simulink model "PannelTest"  (R2022b)
settings: Solver=FixedStepAuto  StartTime=0.0  StopTime=102  FixedStep=0.001  RelTol=1e-3
model workspace (MAT data in the model file):
  Manual_Auto = Simulink.Parameter
  Manual_Auto.Value = 0
  Manual_Auto.DataType = 'auto'
  Manual_Auto.Complexity = 'real'
  Manual_Auto.Dimensions = [1 1]
  Pattern = Simulink.Parameter
  Pattern.Value = 0
  Pattern.DataType = 'auto'
  Pattern.Complexity = 'real'
  Pattern.Dimensions = [1 1]
  Pause_Start = Simulink.Parameter
  Pause_Start.Value = 0
  Pause_Start.DataType = 'auto'
  Pause_Start.Complexity = 'real'
  Pause_Start.Dimensions = [1 1]
  Stop = Simulink.Parameter
  Stop.Value = 0
  Stop.DataType = 'auto'
  Stop.Complexity = 'real'
  Stop.Dimensions = [1 1]
  Unlock_Lock = Simulink.Parameter
  Unlock_Lock.Value = 0
  Unlock_Lock.DataType = 'auto'
  Unlock_Lock.Complexity = 'real'
  Unlock_Lock.Dimensions = [1 1]
undefined symbols (not defined in the file or in its folder): DiscIntNeverNeededParam
(part 1 of 3)
settings Model: Creator=My-Dell-PC  LastModifiedBy=My-Dell-PC

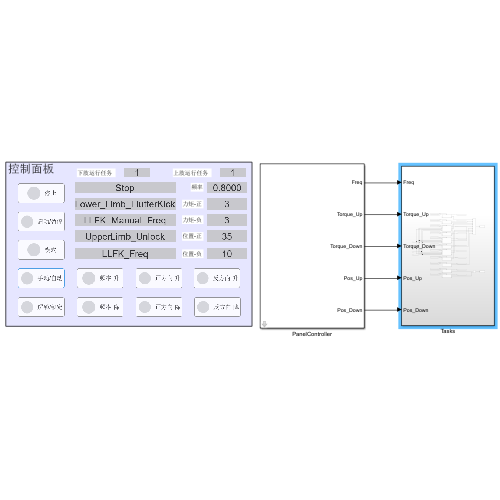
[thumbnail: Simulink's stored preview of the top-level diagram]
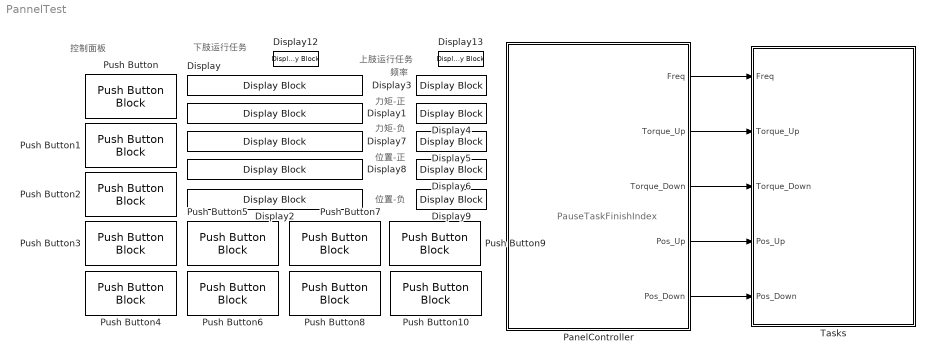
== system PannelTest ==
  note: PauseTaskFinishIndex
  note: 频率
  note: 控制面板
  note: 力矩-正
  note: 力矩-负
  note: 位置-正
  note: 位置-负
  note: 下肢运行任务
  note: 上肢运行任务
  Display{,1..9,12..13} (12 alike) : DisplayBlock  LabelPosition=Hide  Transparency=1
  PanelController : Subsystem  mask{LLFK_Freq_init=0.8, LLB_Freq_init=0.8, LLW_Freq_init=0.8, LLFK_Torque_Up_init=3, LLB_Torque_Up_init=3, LLW_Torque_Up_init=3, LLFK_Torque_Down_init=3, LLB_Torque_Down_init=3, LLW_Torque_Down_init=4.920, LLFK_Pos_Up_init=35, LLB_Pos_Up_init=35, LLW_Pos_Up_init=35, LLFK_Pos_Down_init=10, LLB_Pos_Down_init=10, LLW_Pos_Down_init=10}
      mask prompts: LLFK_Freq_init "LLFK_Freq_init (Hz)"; LLB_Freq_init "LLB_Freq_init (Hz)"; LLW_Freq_init "LLW_Freq_init (Hz)"; LLFK_Torque_Up_init "LLFK_Torque_Up_init (A)"; LLB_Torque_Up_init "LLB_Torque_Up_init (A)"; LLW_Torque_Up_init "LLW_Torque_Up_init (A)"; LLFK_Torque_Down_init "LLFK_Torque_Down_init (A)"; LLB_Torque_Down_init "LLB_Torque_Down_init (A)"; LLW_Torque_Down_init "LLW_Torque_Down_init (A)"; LLFK_Pos_Up_init "LLFK_Pos_Up_init (Degree)"; LLB_Pos_Up_init "LLB_Pos_Up_init (Degree)"; LLW_Pos_Up_init "LLW_Pos_Up_init (Degree)"; LLFK_Pos_Down_init "LLFK_Pos_Down_init (Degree)"; LLB_Pos_Down_init "LLB_Pos_Down_init (Degree)"; LLW_Pos_Down_init "LLW_Pos_Down_init (Degree)"
      mask DialogControl ParameterGroupVar Prompt: Freq_Init
      mask DialogControl Container3 Prompt: Torque_Up_Init
      mask DialogControl Container4 Prompt: Torque_Down_Init
      mask DialogControl Container5 Prompt: Pos_Up_init (Degree)
      mask DialogControl Container6 Prompt: Pos_Down_init (Degree)
  Push Button : PushButtonBlock  ButtonText=停止  Icon=Circle  IconColor=On  OffValue=0.000000
  Push Button1 : PushButtonBlock  ButtonText=启动/暂停  Icon=Circle  IconColor=On  OffValue=0.000000
  Push Button10 : PushButtonBlock  ButtonText=反方向-降  Icon=Circle  IconColor=On  OffValue=0.000000
  Push Button2 : PushButtonBlock  ButtonText=模式  Icon=Circle  IconColor=On  OffValue=0.000000
  Push Button3 : PushButtonBlock  ButtonText=手动/自动  Icon=Circle  IconColor=On  OffValue=0.000000
  Push Button4 : PushButtonBlock  ButtonText=解锁/锁定  Icon=Circle  IconColor=On  OffValue=0.000000
  Push Button5 : PushButtonBlock  ButtonText=频率-升  Icon=Circle  IconColor=On  OffValue=0.000000
  Push Button6 : PushButtonBlock  ButtonText=频率-降  Icon=Circle  IconColor=On  OffValue=0.000000
  Push Button7 : PushButtonBlock  ButtonText=正方向-升  Icon=Circle  IconColor=On  OffValue=0.000000
  Push Button8 : PushButtonBlock  ButtonText=正方向-降  Icon=Circle  IconColor=On  OffValue=0.000000
  Push Button9 : PushButtonBlock  ButtonText=反方向-升  Icon=Circle  IconColor=On  OffValue=0.000000
  Tasks : Subsystem
  wires:
  PanelController/1(Freq) -> Tasks/1(Freq)
  PanelController/2(Torque_Up) -> Tasks/2(Torque_Up)
  PanelController/3(Torque_Down) -> Tasks/3(Torque_Down)
  PanelController/4(Pos_Up) -> Tasks/4(Pos_Up)
  PanelController/5(Pos_Down) -> Tasks/5(Pos_Down)

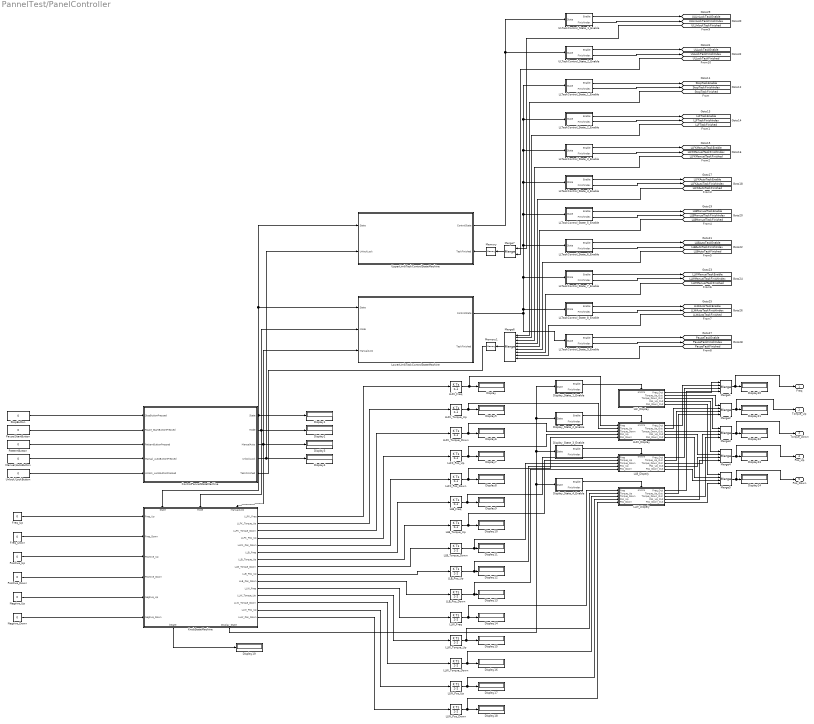
== system PannelTest/PanelController ==
  ControlPannelStateMachine : Stateflow chart  TreatAsAtomicUnit=on
      settings: PortSchema="{\"entries\":[{\"content\":{\"sides\":[{\"content\":{\"connectorIds\":[\"In2\",\"In3\",\"In4\",\"In5\",\"In6\"]},\"type\":\"ConnectorPlacement.EquallySpacedRectSide\",\"uuid\":\"eab411cf-4b6a-48c6-b596-b66f8c420e7c\"},{\"content\":{\"connectorIds\":[\"Out1\",\"Out2\",\"Out3\",\"Out4\",\"In1\"],\"side\":\"RIGHT\"},\"type\":\"ConnectorPlacement.EquallySpacedRectSide\",\"uuid\":\"e0e09f46-7c1c-4140-8220-034119073277\"},{\"content\":{\"connectorIds\":[],\"side\":\"TOP\"},\"type\":\"ConnectorPlacement.EquallySpacedRectSide\",\"uuid\":\"ed6bf201-0ea3-4e7c-82a9-322f02ea728a\"}]},\"type\":\"ConnectorPlacement.EquallySpacedConnector\",\"uuid\":\"aa71b69e-402d-40b0-a3fd-c9400a9adadc\"}],\"packageUris\":[\"http://schema.mathworks.com/mf0/Connector/R2020b\"],\"version\":\"1.0\"}"
  Display{,1..24} (25 alike) : Display
  Display_State_1_Enable : Subsystem  mask{TaskIndex=1}
  Display_State_2_Enable : Subsystem  mask{TaskIndex=2}
  Display_State_3_Enable : Subsystem  mask{TaskIndex=3}
  Display_State_4_Enable : Subsystem  mask{TaskIndex=4}
  Freq_Down : Constant  Value=0
  Freq_Up : Constant  Value=0
  KnobStateMachine : Stateflow chart  TreatAsAtomicUnit=on
      settings: PortSchema="{\"entries\":[{\"content\":{\"sides\":[{\"content\":{\"connectorIds\":[\"In1\",\"In2\",\"In3\",\"In4\",\"In5\",\"In6\"]},\"type\":\"ConnectorPlacement.EquallySpacedRectSide\",\"uuid\":\"78a56fe3-ceb0-42ee-90bc-aa39a12c9afb\"},{\"content\":{\"connectorIds\":[\"Out5\",\"Out3\",\"Out4\",\"Out6\",\"Out7\",\"Out8\",\"Out9\",\"Out10\",\"Out11\",\"Out12\",\"Out13\",\"Out14\",\"Out15\",\"Out16\",\"Out17\"],\"side\":\"RIGHT\"},\"type\":\"ConnectorPlacement.EquallySpacedRectSide\",\"uuid\":\"7553af84-a921-4f96-ace4-e42d4d568d32\"},{\"content\":{\"connectorIds\":[\"In7\",\"In8\",\"In9\"],\"side\":\"TOP\"},\"type\":\"ConnectorPlacement.EquallySpacedRectSide\",\"uuid\":\"299fd0e5-cc5b-4534-8b50-a134eaae2b47\"},{\"content\":{\"connectorIds\":[\"Out1\",\"Out2\"],\"side\":\"BOTTOM\"},\"type\":\"ConnectorPlacement.EquallySpacedRectSide\",\"uuid\":\"12262c62-fe5d-4494-9572-224afcc612c3\"}]},\"type\":\"ConnectorPlacement.EquallySpacedConnector\",\"uuid\":\"b0bd0f4e-3cef-462f-91f5-f8bdfcbb196f\"}],\"packageUris\":[\"http://schema.mathworks.com/mf0/Connector/R2020b\"],\"version\":\"1.0\"}"
  LLB_Dispaly : Subsystem
  LLB_Freq : DiscreteIntegrator  gainval=1000*0.1  InitialCondition=LLB_Freq_init  SampleTime=-1  LimitOutput=on  UpperSaturationLimit=2.5  LowerSaturationLimit=0.3  ICPrevOutput=DiscIntNeverNeededParam  ICPrevScaledInput=DiscIntNeverNeededParam
  LLB_Pos_Down : DiscreteIntegrator  gainval=1000*1  InitialCondition=LLB_Pos_Down_init  SampleTime=-1  LimitOutput=on  UpperSaturationLimit=30  LowerSaturationLimit=5  ICPrevOutput=DiscIntNeverNeededParam  ICPrevScaledInput=DiscIntNeverNeededParam
  LLB_Pos_Up : DiscreteIntegrator  gainval=1000*1  InitialCondition=LLB_Pos_Up_init  SampleTime=-1  LimitOutput=on  UpperSaturationLimit=90  LowerSaturationLimit=10  ICPrevOutput=DiscIntNeverNeededParam  ICPrevScaledInput=DiscIntNeverNeededParam
  LLB_Torque_Down : DiscreteIntegrator  gainval=1000*0.1  InitialCondition=LLB_Torque_Down_init  SampleTime=-1  LimitOutput=on  UpperSaturationLimit=8  LowerSaturationLimit=0  ICPrevOutput=DiscIntNeverNeededParam  ICPrevScaledInput=DiscIntNeverNeededParam
  LLB_Torque_Up : DiscreteIntegrator  gainval=1000*0.1  InitialCondition=LLB_Torque_Up_init  SampleTime=-1  LimitOutput=on  UpperSaturationLimit=8  LowerSaturationLimit=0  ICPrevOutput=DiscIntNeverNeededParam  ICPrevScaledInput=DiscIntNeverNeededParam
  LLFK_Display : Subsystem
  LLFK_Freq : DiscreteIntegrator  gainval=1000*0.1  InitialCondition=LLFK_Freq_init  SampleTime=-1  LimitOutput=on  UpperSaturationLimit=2.5  LowerSaturationLimit=0.3  ICPrevOutput=DiscIntNeverNeededParam  ICPrevScaledInput=DiscIntNeverNeededParam
  LLFK_Pos_Down : DiscreteIntegrator  gainval=1000*1  InitialCondition=LLFK_Pos_Down_init  SampleTime=-1  LimitOutput=on  UpperSaturationLimit=30  LowerSaturationLimit=5  ICPrevOutput=DiscIntNeverNeededParam  ICPrevScaledInput=DiscIntNeverNeededParam
  LLFK_Pos_Up : DiscreteIntegrator  gainval=1000*1  InitialCondition=LLFK_Pos_Up_init  SampleTime=-1  LimitOutput=on  UpperSaturationLimit=90  LowerSaturationLimit=10  ICPrevOutput=DiscIntNeverNeededParam  ICPrevScaledInput=DiscIntNeverNeededParam
  LLFK_Torque_Down : DiscreteIntegrator  gainval=1000*0.1  InitialCondition=LLFK_Torque_Down_init  SampleTime=-1  LimitOutput=on  UpperSaturationLimit=8  LowerSaturationLimit=0  ICPrevOutput=DiscIntNeverNeededParam  ICPrevScaledInput=DiscIntNeverNeededParam
  LLFK_Torque_Up : DiscreteIntegrator  gainval=1000*0.1  InitialCondition=LLFK_Torque_Up_init  SampleTime=-1  LimitOutput=on  UpperSaturationLimit=8  LowerSaturationLimit=0  ICPrevOutput=DiscIntNeverNeededParam  ICPrevScaledInput=DiscIntNeverNeededParam
  LLF_Display : Subsystem
  LLTaskControl_State_1_Enable : Subsystem  mask{TaskIndex=1}
  LLTaskControl_State_2_Enable : Subsystem  mask{TaskIndex=2}
  LLTaskControl_State_3_Enable : Subsystem  mask{TaskIndex=3}
  LLTaskControl_State_4_Enable : Subsystem  mask{TaskIndex=4}
  LLTaskControl_State_5_Enable : Subsystem  mask{TaskIndex=5}
  LLTaskControl_State_6_Enable : Subsystem  mask{TaskIndex=6}
  LLTaskControl_State_7_Enable : Subsystem  mask{TaskIndex=7}
  LLTaskControl_State_8_Enable : Subsystem  mask{TaskIndex=8}
  LLTaskControl_State_9_Enable : Subsystem  mask{TaskIndex=9}
  LLW_Dispaly : Subsystem
  LLW_Freq : DiscreteIntegrator  gainval=1000*0.1  InitialCondition=LLW_Freq_init  SampleTime=-1  LimitOutput=on  UpperSaturationLimit=2.5  LowerSaturationLimit=0.3  ICPrevOutput=DiscIntNeverNeededParam  ICPrevScaledInput=DiscIntNeverNeededParam
  LLW_Pos_Down : DiscreteIntegrator  gainval=1000*1  InitialCondition=LLW_Pos_Down_init  SampleTime=-1  LimitOutput=on  UpperSaturationLimit=30  LowerSaturationLimit=5  ICPrevOutput=DiscIntNeverNeededParam  ICPrevScaledInput=DiscIntNeverNeededParam
  LLW_Pos_Up : DiscreteIntegrator  gainval=1000*1  InitialCondition=LLW_Pos_Up_init  SampleTime=-1  LimitOutput=on  UpperSaturationLimit=90  LowerSaturationLimit=10  ICPrevOutput=DiscIntNeverNeededParam  ICPrevScaledInput=DiscIntNeverNeededParam
  LLW_Torque_Down : DiscreteIntegrator  gainval=1000*0.1  InitialCondition=LLW_Torque_Down_init  SampleTime=-1  LimitOutput=on  UpperSaturationLimit=8  LowerSaturationLimit=0  ICPrevOutput=DiscIntNeverNeededParam  ICPrevScaledInput=DiscIntNeverNeededParam
  LLW_Torque_Up : DiscreteIntegrator  gainval=1000*0.1  InitialCondition=LLW_Torque_Up_init  SampleTime=-1  LimitOutput=on  UpperSaturationLimit=8  LowerSaturationLimit=0  ICPrevOutput=DiscIntNeverNeededParam  ICPrevScaledInput=DiscIntNeverNeededParam
  LowerLimbTaskControlStateMachine : Stateflow chart  TreatAsAtomicUnit=on
      settings: PortSchema="{\"entries\":[{\"content\":{\"sides\":[{\"content\":{\"connectorIds\":[\"In1\",\"In2\",\"In3\"]},\"type\":\"ConnectorPlacement.EquallySpacedRectSide\",\"uuid\":\"03cd27ce-54ab-43c2-a1fd-e45b1fb64ace\"},{\"content\":{\"connectorIds\":[\"Out1\",\"In4\"],\"side\":\"RIGHT\"},\"type\":\"ConnectorPlacement.EquallySpacedRectSide\",\"uuid\":\"abc715eb-7f79-4608-8fec-8488e948793b\"},{\"content\":{\"connectorIds\":[],\"side\":\"TOP\"},\"type\":\"ConnectorPlacement.EquallySpacedRectSide\",\"uuid\":\"1886991b-e2e2-4abe-a6fa-32b2465c841c\"}]},\"type\":\"ConnectorPlacement.EquallySpacedConnector\",\"uuid\":\"4193466d-47aa-4a1d-8728-fb02102c0872\"}],\"packageUris\":[\"http://schema.mathworks.com/mf0/Connector/R2020b\"],\"version\":\"1.0\"}"
  Manual/AutoButton : Constant  Value=0
  Memory : Memory
  Memory1 : Memory
  Merge{1..5} (5 alike) : Merge  Inputs=4
  Merge6 : Merge  Inputs=9
  Merge7 : Merge
  Negtive_Down : Constant  Value=0
  Negtive_Up : Constant  Value=0
  PatternButton : Constant  Value=0
  Pause/StartButton : Constant  Value=0
  Positive_Down : Constant  Value=0
  Positive_Up : Constant  Value=0
  StopButton : Constant  Value=0
  ULTaskControl_State_1_Enable : Subsystem  mask{TaskIndex=1}
  ULTaskControl_State_2_Enable : Subsystem  mask{TaskIndex=2}
  Unlock/LockButton : Constant  Value=0
  UpperLimbTaskControlStateMachine : Stateflow chart  TreatAsAtomicUnit=on
      settings: PortSchema="{\"entries\":[{\"content\":{\"sides\":[{\"content\":{\"connectorIds\":[\"In2\",\"In3\"]},\"type\":\"ConnectorPlacement.EquallySpacedRectSide\",\"uuid\":\"db13f0a7-324e-407f-8bcd-77b68e0b14b1\"},{\"content\":{\"connectorIds\":[\"Out1\",\"In1\"],\"side\":\"RIGHT\"},\"type\":\"ConnectorPlacement.EquallySpacedRectSide\",\"uuid\":\"09ee7819-fd71-4fe3-966c-1072161e5215\"},{\"content\":{\"connectorIds\":[],\"side\":\"TOP\"},\"type\":\"ConnectorPlacement.EquallySpacedRectSide\",\"uuid\":\"7aa19da4-9a31-402b-a0a8-4c1e281f7350\"}]},\"type\":\"ConnectorPlacement.EquallySpacedConnector\",\"uuid\":\"341b49cf-d13f-4e39-8c92-8137a597871d\"}],\"packageUris\":[\"http://schema.mathworks.com/mf0/Connector/R2020b\"],\"version\":\"1.0\"}"
  Freq : Outport
  Torque_Up : Outport  Port=2
  Torque_Down : Outport  Port=3
  Pos_Up : Outport  Port=4
  Pos_Down : Outport  Port=5
  tag scope: LLBAutoTaskEnable=global, LLBAutoTaskFinishIndex=global, LLBManualTaskEnable=global, LLBManualTaskFinishIndex=global, LLFKAutoTaskEnable=global, LLFKAutoTaskFinishIndex=global, LLFKManualTaskEnable=global, LLFKManualTaskFinishIndex=global, LLFTaskEnable=global, LLFTaskFinishIndex=global, LLWAutoTaskEnable=global, LLWAutoTaskFinishIndex=global, LLWManualTaskEnable=global, LLWManualTaskFinishIndex=global, PauseTaskEnable=global, PauseTaskFinishIndex=global, StopTaskEnable=global, StopTaskFinishIndex=global, ULLockTaskEnable=global, ULLockTaskFinishIndex=global, ULUnLockTaskEnable=global, ULUnLockTaskFinishIndex=global
  wires:
  StopButton/1 -> ControlPannelStateMachine/2(StopButtonPressed)
  ControlPannelStateMachine/1(State) -> UpperLimbTaskControlStateMachine/2(State), LowerLimbTaskControlStateMachine/1(State), Display1/1, KnobStateMachine/7(State)
  Pause/StartButton/1 -> ControlPannelStateMachine/3(Pause_StartButtonPressed)
  PatternButton/1 -> ControlPannelStateMachine/4(PatternButtonPressed)
  Manual/AutoButton/1 -> ControlPannelStateMachine/5(Manual_AutoButtonPressed)
  ControlPannelStateMachine/2(Mode) -> KnobStateMachine/8(Mode), Display2/1, LowerLimbTaskControlStateMachine/2(Mode)
  ControlPannelStateMachine/3(ManualAuto) -> KnobStateMachine/9(ManualAuto), Display3/1, LowerLimbTaskControlStateMachine/3(ManualAuto)
  Unlock/LockButton/1 -> ControlPannelStateMachine/6(Unlock_LockButtonPressed)
  ControlPannelStateMachine/4(UnlockLock) -> Display4/1, UpperLimbTaskControlStateMachine/3(UnlockLock)
  LLFK_Freq/1 -> LLFK_Display/1(Freq), Display/1
  LLFK_Pos_Down/1 -> LLFK_Display/5(Pos_Down), Display8/1
  LLFK_Pos_Up/1 -> LLFK_Display/4(Pos_Up), Display7/1
  LLFK_Torque_Down/1 -> LLFK_Display/3(Torque_Down), Display6/1
  LLFK_Torque_Up/1 -> LLFK_Display/2(Torque_Up), Display5/1
  KnobStateMachine/5(LLFK_Freq) -> LLFK_Freq/1
  KnobStateMachine/3(LLFK_Torque_Up) -> LLFK_Torque_Up/1
  KnobStateMachine/4(LLFK_Torque_Down) -> LLFK_Torque_Down/1
  KnobStateMachine/6(LLFK_Pos_Up) -> LLFK_Pos_Up/1
  KnobStateMachine/7(LLFK_Pos_Down) -> LLFK_Pos_Down/1
  Freq_Up/1 -> KnobStateMachine/1(Freq_Up)
  Freq_Down/1 -> KnobStateMachine/2(Freq_Down)
  Positive_Up/1 -> KnobStateMachine/3(Positive_Up)
  Positive_Down/1 -> KnobStateMachine/4(Positive_Down)
  Negtive_Up/1 -> KnobStateMachine/5(Negtive_Up)
  Negtive_Down/1 -> KnobStateMachine/6(Negtive_Down)
  KnobStateMachine/9(LLB_Torque_Up) -> LLB_Torque_Up/1
  LLB_Pos_Up/1 -> LLB_Dispaly/4(Pos_Up), Display12/1
  KnobStateMachine/11(LLB_Pos_Up) -> LLB_Pos_Up/1
  LLB_Torque_Down/1 -> Display11/1, LLB_Dispaly/3(Torque_Down)
  LLB_Pos_Down/1 -> LLB_Dispaly/5(Pos_Down), Display13/1
  KnobStateMachine/10(LLB_Torque_Down) -> LLB_Torque_Down/1
  KnobStateMachine/12(LLB_Pos_Down) -> LLB_Pos_Down/1
  LLB_Freq/1 -> LLB_Dispaly/1(Freq), Display9/1
  LLB_Torque_Up/1 -> Display10/1, LLB_Dispaly/2(Torque_Up)
  KnobStateMachine/8(LLB_Freq) -> LLB_Freq/1
  KnobStateMachine/14(LLW_Torque_Up) -> LLW_Torque_Up/1
  LLW_Pos_Up/1 -> LLW_Dispaly/4(Pos_Up), Display17/1
  KnobStateMachine/16(LLW_Pos_Up) -> LLW_Pos_Up/1
  LLW_Torque_Down/1 -> LLW_Dispaly/3(Torque_Down), Display16/1
  KnobStateMachine/15(LLW_Torque_Down) -> LLW_Torque_Down/1
  KnobStateMachine/17(LLW_Pos_Down) -> LLW_Pos_Down/1
  LLW_Freq/1 -> LLW_Dispaly/1(Freq), Display14/1
  KnobStateMachine/13(LLW_Freq) -> LLW_Freq/1
  LLW_Torque_Up/1 -> LLW_Dispaly/2(Torque_Up), Display15/1
  LLW_Pos_Down/1 -> LLW_Dispaly/5(Pos_Down), Display18/1
  KnobStateMachine/1(kState) -> Display19/1
  Display_State_1_Enable/1(Enable) -> LLF_Display/Enable
  Display_State_2_Enable/1(Enable) -> LLFK_Display/Enable
  Display_State_3_Enable/1(Enable) -> LLB_Dispaly/Enable
  Display_State_4_Enable/1(Enable) -> LLW_Dispaly/Enable
  Merge1/1 -> Freq/1, Display20/1
  Merge2/1 -> Torque_Up/1, Display21/1
  Merge3/1 -> Torque_Down/1, Display22/1
  Merge4/1 -> Pos_Up/1, Display23/1
  Merge5/1 -> Pos_Down/1, Display24/1
  KnobStateMachine/2(Display_State) -> Display_State_1_Enable/1(State), Display_State_2_Enable/1(State), Display_State_3_Enable/1(State), Display_State_4_Enable/1(State)
  LLF_Display/1(Freq_Out) -> Merge1/1
  LLFK_Display/1(Freq_Out) -> Merge1/2
  LLB_Dispaly/1(Freq_Out) -> Merge1/3
  LLW_Dispaly/1(Freq_Out) -> Merge1/4
  LLF_Display/2(Torque_Up_Out) -> Merge2/1
  LLFK_Display/2(Torque_Up_Out) -> Merge2/2
  LLB_Dispaly/2(Torque_Up_Out) -> Merge2/3
  LLW_Dispaly/2(Torque_Up_Out) -> Merge2/4
  LLF_Display/3(Torque_Down_Out) -> Merge3/1
  LLFK_Display/3(Torque_Down_Out) -> Merge3/2
  LLB_Dispaly/3(Torque_Down_Out) -> Merge3/3
  LLW_Dispaly/3(Torque_Down_Out) -> Merge3/4
  LLF_Display/4(Pos_Up_Out) -> Merge4/1
  LLFK_Display/4(Pos_Up_Out) -> Merge4/2
  LLB_Dispaly/4(Pos_Up_Out) -> Merge4/3
  LLW_Dispaly/4(Pos_Up_Out) -> Merge4/4
  LLF_Display/5(Pos_Down_Out) -> Merge5/1
  LLFK_Display/5(Pos_Down_Out) -> Merge5/2
  LLB_Dispaly/5(Pos_Down_Out) -> Merge5/3
  LLW_Dispaly/5(Pos_Down_Out) -> Merge5/4
  [StopTaskFinished] -> Merge6/1
  LowerLimbTaskControlStateMachine/1(ControlState) -> LLTaskControl_State_9_Enable/1(State), LLTaskControl_State_1_Enable/1(State), LLTaskControl_State_2_Enable/1(State), LLTaskControl_State_3_Enable/1(State), LLTaskControl_State_4_Enable/1(State), LLTaskControl_State_5_Enable/1(State), LLTaskControl_State_6_Enable/1(State), LLTaskControl_State_7_Enable/1(State), LLTaskControl_State_8_Enable/1(State)
  Merge6/1 -> Memory1/1
  [LLFTaskFinished] -> Merge6/2
  [LLFKManualTaskFinished] -> Merge6/3
  [LLBManualTaskFinished] -> Merge6/5
  [LLWManualTaskFinished] -> Merge6/7
  [PauseTaskFinished] -> Merge6/9
  [LLFKAutoTaskFinished] -> Merge6/4
  [LLBAutoTaskFinished] -> Merge6/6
  [LLWAutoTaskFinished] -> Merge6/8
  Merge7/1 -> Memory/1
  [ULUnlockTaskFinished] -> Merge7/1
  [ULLockTaskFinished] -> Merge7/2
  UpperLimbTaskControlStateMachine/1(ControlState) -> ULTaskControl_State_2_Enable/1(State), ULTaskControl_State_1_Enable/1(State)
  LLTaskControl_State_8_Enable/1(Enable) -> [LLWAutoTaskEnable]
  LLTaskControl_State_5_Enable/2(FinishIndex) -> [LLBManualTaskFinishIndex]
  LLTaskControl_State_8_Enable/2(FinishIndex) -> [LLWAutoTaskFinishIndex]
  LLTaskControl_State_7_Enable/2(FinishIndex) -> [LLWManualTaskFinishIndex]
  LLTaskControl_State_1_Enable/2(FinishIndex) -> [StopTaskFinishIndex]
  LLTaskControl_State_3_Enable/1(Enable) -> [LLFKManualTaskEnable]
  ULTaskControl_State_2_Enable/1(Enable) -> [ULLockTaskEnable]
  LLTaskControl_State_4_Enable/1(Enable) -> [LLFKAutoTaskEnable]
  ULTaskControl_State_1_Enable/2(FinishIndex) -> [ULUnLockTaskFinishIndex]
  LLTaskControl_State_9_Enable/1(Enable) -> [PauseTaskEnable]
  LLTaskControl_State_9_Enable/2(FinishIndex) -> [PauseTaskFinishIndex]
  LLTaskControl_State_3_Enable/2(FinishIndex) -> [LLFKManualTaskFinishIndex]
  LLTaskControl_State_4_Enable/2(FinishIndex) -> [LLFKAutoTaskFinishIndex]
  LLTaskControl_State_5_Enable/1(Enable) -> [LLBManualTaskEnable]
  LLTaskControl_State_2_Enable/1(Enable) -> [LLFTaskEnable]
  LLTaskControl_State_2_Enable/2(FinishIndex) -> [LLFTaskFinishIndex]
  LLTaskControl_State_1_Enable/1(Enable) -> [StopTaskEnable]
  LLTaskControl_State_6_Enable/2(FinishIndex) -> [LLBAutoTaskFinishIndex]
  LLTaskControl_State_6_Enable/1(Enable) -> [LLBAutoTaskEnable]
  ULTaskControl_State_2_Enable/2(FinishIndex) -> [ULLockTaskFinishIndex]
  LLTaskControl_State_7_Enable/1(Enable) -> [LLWManualTaskEnable]
  ULTaskControl_State_1_Enable/1(Enable) -> [ULUnLockTaskEnable]
  Memory/1 -> UpperLimbTaskControlStateMachine/1(TaskFinished)
  Memory1/1 -> ControlPannelStateMachine/1(TaskFinished)

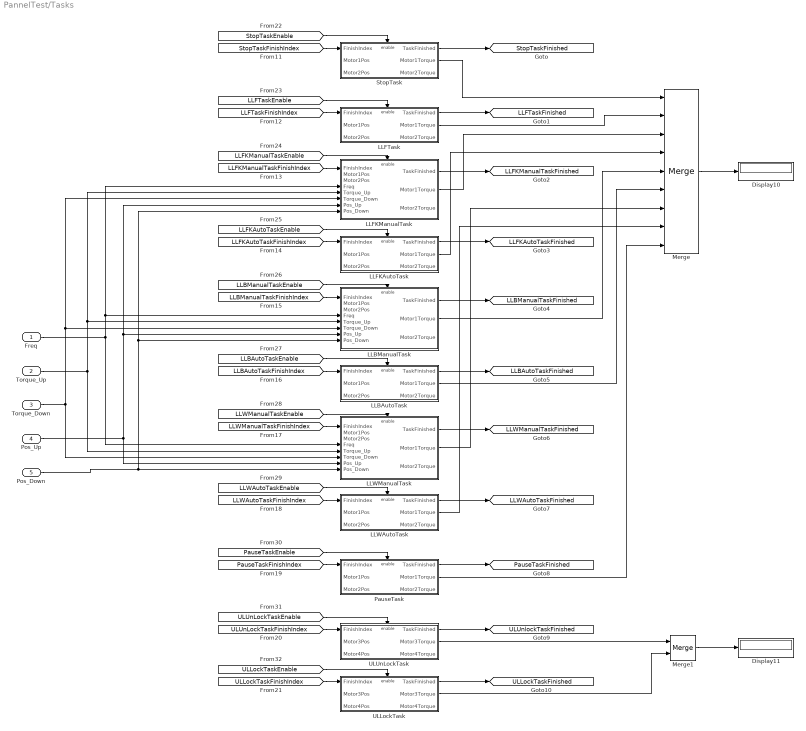
== system PannelTest/Tasks ==
  Freq : Inport
  Torque_Up : Inport  Port=2
  Torque_Down : Inport  Port=3
  Pos_Up : Inport  Port=4
  Pos_Down : Inport  Port=5
  Display10 : Display
  Display11 : Display
  LLBAutoTask : Subsystem
  LLBManualTask : Subsystem
  LLFKAutoTask : Subsystem
  LLFKManualTask : Subsystem
  LLFTask : Subsystem
  LLWAutoTask : Subsystem
  LLWManualTask : Subsystem
  Merge : Merge  Inputs=9
  Merge1 : Merge
  PauseTask : Subsystem
  StopTask : Subsystem
  ULLockTask : Subsystem
  ULUnLockTask : Subsystem
  tag scope: LLBAutoTaskFinished=global, LLBManualTaskFinished=global, LLFKAutoTaskFinished=global, LLFKManualTaskFinished=global, LLFTaskFinished=global, LLWAutoTaskFinished=global, LLWManualTaskFinished=global, PauseTaskFinished=global, StopTaskFinished=global, ULLockTaskFinished=global, ULUnlockTaskFinished=global
  wires:
  ULLockTask/2(Motor3Torque) -> Merge1/2
  LLFKAutoTask/2(Motor1Torque) -> Merge/4
  LLFKManualTask/1(TaskFinished) -> [LLFKManualTaskFinished]
  [ULLockTaskFinishIndex] -> ULLockTask/1(FinishIndex)
  [ULUnLockTaskFinishIndex] -> ULUnLockTask/1(FinishIndex)
  Torque_Up/1 -> LLFKManualTask/5(Torque_Up), LLBManualTask/5(Torque_Up), LLWManualTask/5(Torque_Up)
  Pos_Down/1 -> LLWManualTask/8(Pos_Down), LLBManualTask/8(Pos_Down), LLFKManualTask/8(Pos_Down)
  ULUnLockTask/2(Motor3Torque) -> Merge1/1
  LLWAutoTask/2(Motor1Torque) -> Merge/8
  [LLBAutoTaskEnable] -> LLBAutoTask/Enable
  [LLBManualTaskFinishIndex] -> LLBManualTask/1(FinishIndex)
  [LLFKAutoTaskFinishIndex] -> LLFKAutoTask/1(FinishIndex)
  [LLFTaskEnable] -> LLFTask/Enable
  [ULLockTaskEnable] -> ULLockTask/Enable
  LLBManualTask/1(TaskFinished) -> [LLBManualTaskFinished]
  PauseTask/1(TaskFinished) -> [PauseTaskFinished]
  [LLBManualTaskEnable] -> LLBManualTask/Enable
  Merge/1 -> Display10/1
  Freq/1 -> LLBManualTask/4(Freq), LLFKManualTask/4(Freq), LLWManualTask/4(Freq)
  [LLFKManualTaskFinishIndex] -> LLFKManualTask/1(FinishIndex)
  PauseTask/2(Motor1Torque) -> Merge/9
  Torque_Down/1 -> LLFKManualTask/6(Torque_Down), LLBManualTask/6(Torque_Down), LLWManualTask/6(Torque_Down)
  LLBManualTask/2(Motor1Torque) -> Merge/5
  ULLockTask/1(TaskFinished) -> [ULLockTaskFinished]
  [StopTaskEnable] -> StopTask/Enable
  LLFTask/2(Motor1Torque) -> Merge/2
  [PauseTaskFinishIndex] -> PauseTask/1(FinishIndex)
  LLWManualTask/1(TaskFinished) -> [LLWManualTaskFinished]
  Merge1/1 -> Display11/1
  LLFKAutoTask/1(TaskFinished) -> [LLFKAutoTaskFinished]
  [LLFKAutoTaskEnable] -> LLFKAutoTask/Enable
  [LLWManualTaskEnable] -> LLWManualTask/Enable
  Pos_Up/1 -> LLWManualTask/7(Pos_Up), LLBManualTask/7(Pos_Up), LLFKManualTask/7(Pos_Up)
  ULUnLockTask/1(TaskFinished) -> [ULUnlockTaskFinished]
  [LLWAutoTaskFinishIndex] -> LLWAutoTask/1(FinishIndex)
  [LLBAutoTaskFinishIndex] -> LLBAutoTask/1(FinishIndex)
  [LLWAutoTaskEnable] -> LLWAutoTask/Enable
  StopTask/1(TaskFinished) -> [StopTaskFinished]
  [LLFTaskFinishIndex] -> LLFTask/1(FinishIndex)
  LLFKManualTask/2(Motor1Torque) -> Merge/3
  LLBAutoTask/2(Motor1Torque) -> Merge/6
  LLFTask/1(TaskFinished) -> [LLFTaskFinished]
  [PauseTaskEnable] -> PauseTask/Enable
  [ULUnLockTaskEnable] -> ULUnLockTask/Enable
  [StopTaskFinishIndex] -> StopTask/1(FinishIndex)
  [LLFKManualTaskEnable] -> LLFKManualTask/Enable
  LLWManualTask/2(Motor1Torque) -> Merge/7
  LLBAutoTask/1(TaskFinished) -> [LLBAutoTaskFinished]
  LLWAutoTask/1(TaskFinished) -> [LLWAutoTaskFinished]
  [LLWManualTaskFinishIndex] -> LLWManualTask/1(FinishIndex)
  StopTask/2(Motor1Torque) -> Merge/1

== system PannelTest/PanelController/Display_State_1_Enable ==
  State : Inport
  Subsystem : Subsystem
  Switch Case : SwitchCase  CaseConditions={TaskIndex}
  Enable : Outport
  FinishIndex : Outport  Port=2
  wires:
  Switch Case/2 -> Subsystem/2(Case Default)
  Switch Case/1 -> Subsystem/1(Case)
  Subsystem/2(FinishIndex) -> FinishIndex/1
  Subsystem/1(Enable) -> Enable/1
  State/1 -> Switch Case/1

== system PannelTest/PanelController/Display_State_2_Enable ==
  State : Inport
  Subsystem : Subsystem
  Switch Case : SwitchCase  CaseConditions={TaskIndex}
  Enable : Outport
  FinishIndex : Outport  Port=2
  wires:
  Switch Case/2 -> Subsystem/2(Case Default)
  Switch Case/1 -> Subsystem/1(Case)
  Subsystem/2(FinishIndex) -> FinishIndex/1
  Subsystem/1(Enable) -> Enable/1
  State/1 -> Switch Case/1

== system PannelTest/PanelController/Display_State_3_Enable ==
  State : Inport
  Subsystem : Subsystem
  Switch Case : SwitchCase  CaseConditions={TaskIndex}
  Enable : Outport
  FinishIndex : Outport  Port=2
  wires:
  Switch Case/2 -> Subsystem/2(Case Default)
  Switch Case/1 -> Subsystem/1(Case)
  Subsystem/2(FinishIndex) -> FinishIndex/1
  Subsystem/1(Enable) -> Enable/1
  State/1 -> Switch Case/1

== system PannelTest/PanelController/Display_State_4_Enable ==
  State : Inport
  Subsystem : Subsystem
  Switch Case : SwitchCase  CaseConditions={TaskIndex}
  Enable : Outport
  FinishIndex : Outport  Port=2
  wires:
  Switch Case/2 -> Subsystem/2(Case Default)
  Switch Case/1 -> Subsystem/1(Case)
  Subsystem/2(FinishIndex) -> FinishIndex/1
  Subsystem/1(Enable) -> Enable/1
  State/1 -> Switch Case/1

== system PannelTest/PanelController/LLB_Dispaly ==
  Freq : Inport
  Torque_Up : Inport  Port=2
  Torque_Down : Inport  Port=3
  Pos_Up : Inport  Port=4
  Pos_Down : Inport  Port=5
  Enable : EnablePort
  Freq_Out : Outport
  Torque_Up_Out : Outport  Port=2
  Torque_Down_Out : Outport  Port=3
  Pos_Up_Out : Outport  Port=4
  Pos_Down_Out : Outport  Port=5
  wires:
  Freq/1 -> Freq_Out/1
  Torque_Up/1 -> Torque_Up_Out/1
  Torque_Down/1 -> Torque_Down_Out/1
  Pos_Up/1 -> Pos_Up_Out/1
  Pos_Down/1 -> Pos_Down_Out/1

== system PannelTest/PanelController/LLFK_Display ==
  Freq : Inport
  Torque_Up : Inport  Port=2
  Torque_Down : Inport  Port=3
  Pos_Up : Inport  Port=4
  Pos_Down : Inport  Port=5
  Enable : EnablePort
  Freq_Out : Outport
  Torque_Up_Out : Outport  Port=2
  Torque_Down_Out : Outport  Port=3
  Pos_Up_Out : Outport  Port=4
  Pos_Down_Out : Outport  Port=5
  wires:
  Freq/1 -> Freq_Out/1
  Torque_Up/1 -> Torque_Up_Out/1
  Torque_Down/1 -> Torque_Down_Out/1
  Pos_Up/1 -> Pos_Up_Out/1
  Pos_Down/1 -> Pos_Down_Out/1

== system PannelTest/PanelController/LLF_Display ==
  Enable : EnablePort
  Constant{,1..4} (5 alike) : Constant  Value=0
  Freq_Out : Outport
  Torque_Up_Out : Outport  Port=2
  Torque_Down_Out : Outport  Port=3
  Pos_Up_Out : Outport  Port=4
  Pos_Down_Out : Outport  Port=5
  wires:
  Constant/1 -> Freq_Out/1
  Constant1/1 -> Torque_Up_Out/1
  Constant2/1 -> Torque_Down_Out/1
  Constant3/1 -> Pos_Up_Out/1
  Constant4/1 -> Pos_Down_Out/1

== system PannelTest/PanelController/LLTaskControl_State_1_Enable ==
  State : Inport
  Subsystem : Subsystem
  Switch Case : SwitchCase  CaseConditions={TaskIndex}
  Enable : Outport
  FinishIndex : Outport  Port=2
  wires:
  Switch Case/2 -> Subsystem/2(Case Default)
  Switch Case/1 -> Subsystem/1(Case)
  Subsystem/2(FinishIndex) -> FinishIndex/1
  Subsystem/1(Enable) -> Enable/1
  State/1 -> Switch Case/1

== system PannelTest/PanelController/LLTaskControl_State_2_Enable ==
  State : Inport
  Subsystem : Subsystem
  Switch Case : SwitchCase  CaseConditions={TaskIndex}
  Enable : Outport
  FinishIndex : Outport  Port=2
  wires:
  Switch Case/2 -> Subsystem/2(Case Default)
  Switch Case/1 -> Subsystem/1(Case)
  Subsystem/2(FinishIndex) -> FinishIndex/1
  Subsystem/1(Enable) -> Enable/1
  State/1 -> Switch Case/1

== system PannelTest/PanelController/LLTaskControl_State_3_Enable ==
  State : Inport
  Subsystem : Subsystem
  Switch Case : SwitchCase  CaseConditions={TaskIndex}
  Enable : Outport
  FinishIndex : Outport  Port=2
  wires:
  Switch Case/2 -> Subsystem/2(Case Default)
  Switch Case/1 -> Subsystem/1(Case)
  Subsystem/2(FinishIndex) -> FinishIndex/1
  Subsystem/1(Enable) -> Enable/1
  State/1 -> Switch Case/1

== system PannelTest/PanelController/LLTaskControl_State_4_Enable ==
  State : Inport
  Subsystem : Subsystem
  Switch Case : SwitchCase  CaseConditions={TaskIndex}
  Enable : Outport
  FinishIndex : Outport  Port=2
  wires:
  Switch Case/2 -> Subsystem/2(Case Default)
  Switch Case/1 -> Subsystem/1(Case)
  Subsystem/2(FinishIndex) -> FinishIndex/1
  Subsystem/1(Enable) -> Enable/1
  State/1 -> Switch Case/1

== system PannelTest/PanelController/LLTaskControl_State_5_Enable ==
  State : Inport
  Subsystem : Subsystem
  Switch Case : SwitchCase  CaseConditions={TaskIndex}
  Enable : Outport
  FinishIndex : Outport  Port=2
  wires:
  Switch Case/2 -> Subsystem/2(Case Default)
  Switch Case/1 -> Subsystem/1(Case)
  Subsystem/2(FinishIndex) -> FinishIndex/1
  Subsystem/1(Enable) -> Enable/1
  State/1 -> Switch Case/1

== system PannelTest/PanelController/LLTaskControl_State_6_Enable ==
  State : Inport
  Subsystem : Subsystem
  Switch Case : SwitchCase  CaseConditions={TaskIndex}
  Enable : Outport
  FinishIndex : Outport  Port=2
  wires:
  Switch Case/2 -> Subsystem/2(Case Default)
  Switch Case/1 -> Subsystem/1(Case)
  Subsystem/2(FinishIndex) -> FinishIndex/1
  Subsystem/1(Enable) -> Enable/1
  State/1 -> Switch Case/1

== system PannelTest/PanelController/LLTaskControl_State_7_Enable ==
  State : Inport
  Subsystem : Subsystem
  Switch Case : SwitchCase  CaseConditions={TaskIndex}
  Enable : Outport
  FinishIndex : Outport  Port=2
  wires:
  Switch Case/2 -> Subsystem/2(Case Default)
  Switch Case/1 -> Subsystem/1(Case)
  Subsystem/2(FinishIndex) -> FinishIndex/1
  Subsystem/1(Enable) -> Enable/1
  State/1 -> Switch Case/1

== system PannelTest/PanelController/LLTaskControl_State_8_Enable ==
  State : Inport
  Subsystem : Subsystem
  Switch Case : SwitchCase  CaseConditions={TaskIndex}
  Enable : Outport
  FinishIndex : Outport  Port=2
  wires:
  Switch Case/2 -> Subsystem/2(Case Default)
  Switch Case/1 -> Subsystem/1(Case)
  Subsystem/2(FinishIndex) -> FinishIndex/1
  Subsystem/1(Enable) -> Enable/1
  State/1 -> Switch Case/1

== system PannelTest/PanelController/LLTaskControl_State_9_Enable ==
  State : Inport
  Subsystem : Subsystem
  Switch Case : SwitchCase  CaseConditions={TaskIndex}
  Enable : Outport
  FinishIndex : Outport  Port=2
  wires:
  Switch Case/2 -> Subsystem/2(Case Default)
  Switch Case/1 -> Subsystem/1(Case)
  Subsystem/2(FinishIndex) -> FinishIndex/1
  Subsystem/1(Enable) -> Enable/1
  State/1 -> Switch Case/1

== system PannelTest/PanelController/LLW_Dispaly ==
  Freq : Inport
  Torque_Up : Inport  Port=2
  Torque_Down : Inport  Port=3
  Pos_Up : Inport  Port=4
  Pos_Down : Inport  Port=5
  Enable : EnablePort
  Freq_Out : Outport
  Torque_Up_Out : Outport  Port=2
  Torque_Down_Out : Outport  Port=3
  Pos_Up_Out : Outport  Port=4
  Pos_Down_Out : Outport  Port=5
  wires:
  Freq/1 -> Freq_Out/1
  Torque_Up/1 -> Torque_Up_Out/1
  Torque_Down/1 -> Torque_Down_Out/1
  Pos_Up/1 -> Pos_Up_Out/1
  Pos_Down/1 -> Pos_Down_Out/1

== system PannelTest/PanelController/ULTaskControl_State_1_Enable ==
  State : Inport
  Subsystem : Subsystem
  Switch Case : SwitchCase  CaseConditions={TaskIndex}
  Enable : Outport
  FinishIndex : Outport  Port=2
  wires:
  Switch Case/2 -> Subsystem/2(Case Default)
  Switch Case/1 -> Subsystem/1(Case)
  Subsystem/2(FinishIndex) -> FinishIndex/1
  Subsystem/1(Enable) -> Enable/1
  State/1 -> Switch Case/1

== system PannelTest/PanelController/ULTaskControl_State_2_Enable ==
  State : Inport
  Subsystem : Subsystem
  Switch Case : SwitchCase  CaseConditions={TaskIndex}
  Enable : Outport
  FinishIndex : Outport  Port=2
  wires:
  Switch Case/2 -> Subsystem/2(Case Default)
  Switch Case/1 -> Subsystem/1(Case)
  Subsystem/2(FinishIndex) -> FinishIndex/1
  Subsystem/1(Enable) -> Enable/1
  State/1 -> Switch Case/1

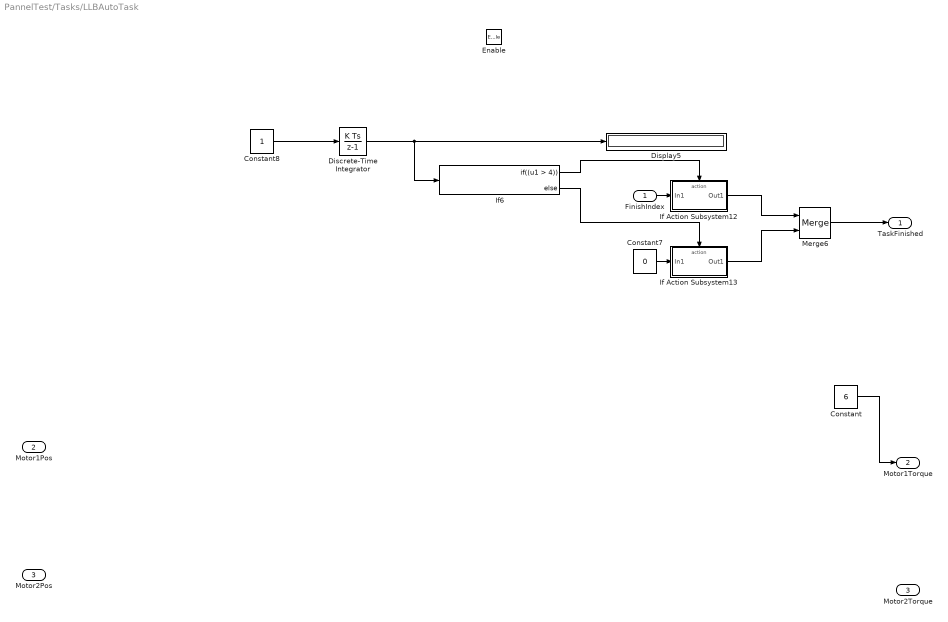
== system PannelTest/Tasks/LLBAutoTask ==
  FinishIndex : Inport
  Motor1Pos : Inport  Port=2
  Motor2Pos : Inport  Port=3
  Enable : EnablePort  StatesWhenEnabling=reset
  Constant : Constant  Value=6
  Constant7 : Constant  Value=0  OutDataTypeStr=double
  Constant8 : Constant
  Discrete-Time Integrator : DiscreteIntegrator  SampleTime=-1  ICPrevOutput=DiscIntNeverNeededParam  ICPrevScaledInput=DiscIntNeverNeededParam
  Display5 : Display
  If Action Subsystem12 : Subsystem  TreatAsAtomicUnit=on
  If Action Subsystem13 : Subsystem  TreatAsAtomicUnit=on
  If6 : If  IfExpression=(u1 > 4)
  Merge6 : Merge
  TaskFinished : Outport
  Motor1Torque : Outport  Port=2
  Motor2Torque : Outport  Port=3
  wires:
  Merge6/1 -> TaskFinished/1
  If6/1 -> If Action Subsystem12/Action
  Constant8/1 -> Discrete-Time Integrator/1
  If6/2 -> If Action Subsystem13/Action
  Discrete-Time Integrator/1 -> If6/1, Display5/1
  If Action Subsystem13/1(Out1) -> Merge6/2
  FinishIndex/1 -> If Action Subsystem12/1(In1)
  If Action Subsystem12/1(Out1) -> Merge6/1
  Constant7/1 -> If Action Subsystem13/1(In1)
  Constant/1 -> Motor1Torque/1

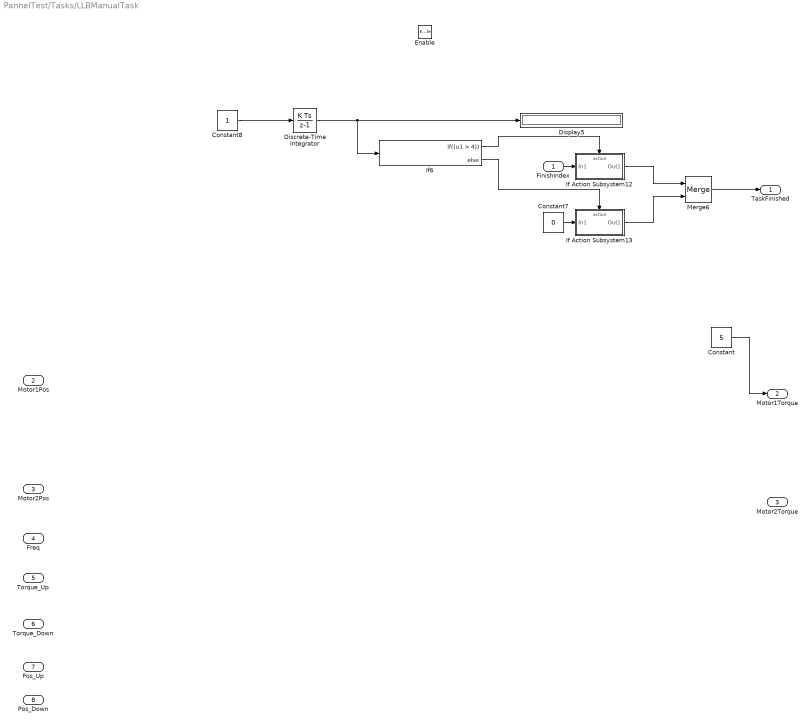
== system PannelTest/Tasks/LLBManualTask ==
  FinishIndex : Inport
  Motor1Pos : Inport  Port=2
  Motor2Pos : Inport  Port=3
  Freq : Inport  Port=4
  Torque_Up : Inport  Port=5
  Torque_Down : Inport  Port=6
  Pos_Up : Inport  Port=7
  Pos_Down : Inport  Port=8
  Enable : EnablePort  StatesWhenEnabling=reset
  Constant : Constant  Value=5
  Constant7 : Constant  Value=0  OutDataTypeStr=double
  Constant8 : Constant
  Discrete-Time Integrator : DiscreteIntegrator  SampleTime=-1  ICPrevOutput=DiscIntNeverNeededParam  ICPrevScaledInput=DiscIntNeverNeededParam
  Display5 : Display
  If Action Subsystem12 : Subsystem  TreatAsAtomicUnit=on
  If Action Subsystem13 : Subsystem  TreatAsAtomicUnit=on
  If6 : If  IfExpression=(u1 > 4)
  Merge6 : Merge
  TaskFinished : Outport
  Motor1Torque : Outport  Port=2
  Motor2Torque : Outport  Port=3
  wires:
  Merge6/1 -> TaskFinished/1
  If6/1 -> If Action Subsystem12/Action
  Constant8/1 -> Discrete-Time Integrator/1
  If6/2 -> If Action Subsystem13/Action
  Discrete-Time Integrator/1 -> If6/1, Display5/1
  If Action Subsystem13/1(Out1) -> Merge6/2
  FinishIndex/1 -> If Action Subsystem12/1(In1)
  If Action Subsystem12/1(Out1) -> Merge6/1
  Constant7/1 -> If Action Subsystem13/1(In1)
  Constant/1 -> Motor1Torque/1

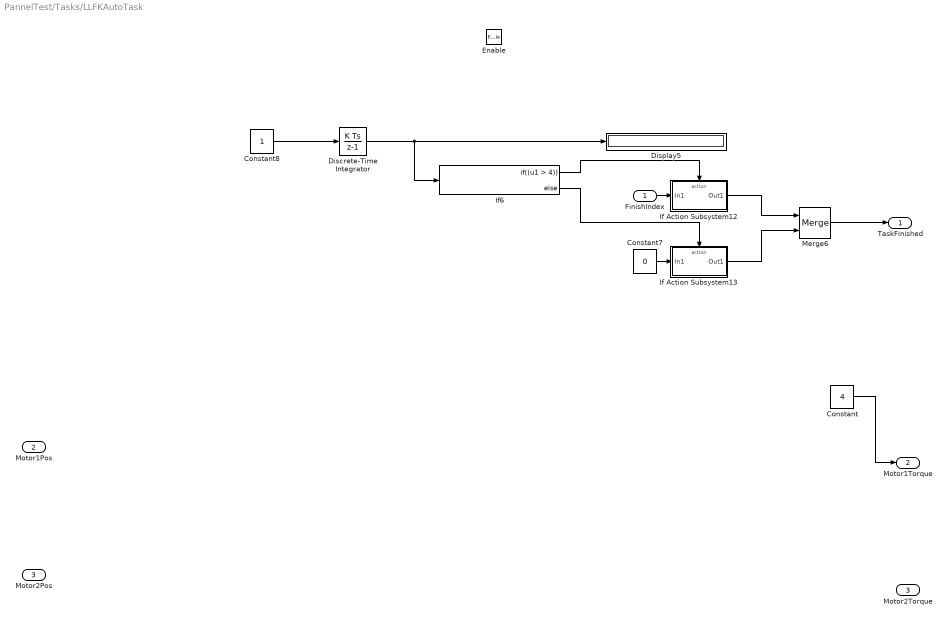
== system PannelTest/Tasks/LLFKAutoTask ==
  FinishIndex : Inport
  Motor1Pos : Inport  Port=2
  Motor2Pos : Inport  Port=3
  Enable : EnablePort  StatesWhenEnabling=reset
  Constant : Constant  Value=4
  Constant7 : Constant  Value=0  OutDataTypeStr=double
  Constant8 : Constant
  Discrete-Time Integrator : DiscreteIntegrator  SampleTime=-1  ICPrevOutput=DiscIntNeverNeededParam  ICPrevScaledInput=DiscIntNeverNeededParam
  Display5 : Display
  If Action Subsystem12 : Subsystem  TreatAsAtomicUnit=on
  If Action Subsystem13 : Subsystem  TreatAsAtomicUnit=on
  If6 : If  IfExpression=(u1 > 4)
  Merge6 : Merge
  TaskFinished : Outport
  Motor1Torque : Outport  Port=2
  Motor2Torque : Outport  Port=3
  wires:
  Merge6/1 -> TaskFinished/1
  If6/1 -> If Action Subsystem12/Action
  Constant8/1 -> Discrete-Time Integrator/1
  If6/2 -> If Action Subsystem13/Action
  Discrete-Time Integrator/1 -> If6/1, Display5/1
  If Action Subsystem13/1(Out1) -> Merge6/2
  FinishIndex/1 -> If Action Subsystem12/1(In1)
  If Action Subsystem12/1(Out1) -> Merge6/1
  Constant7/1 -> If Action Subsystem13/1(In1)
  Constant/1 -> Motor1Torque/1

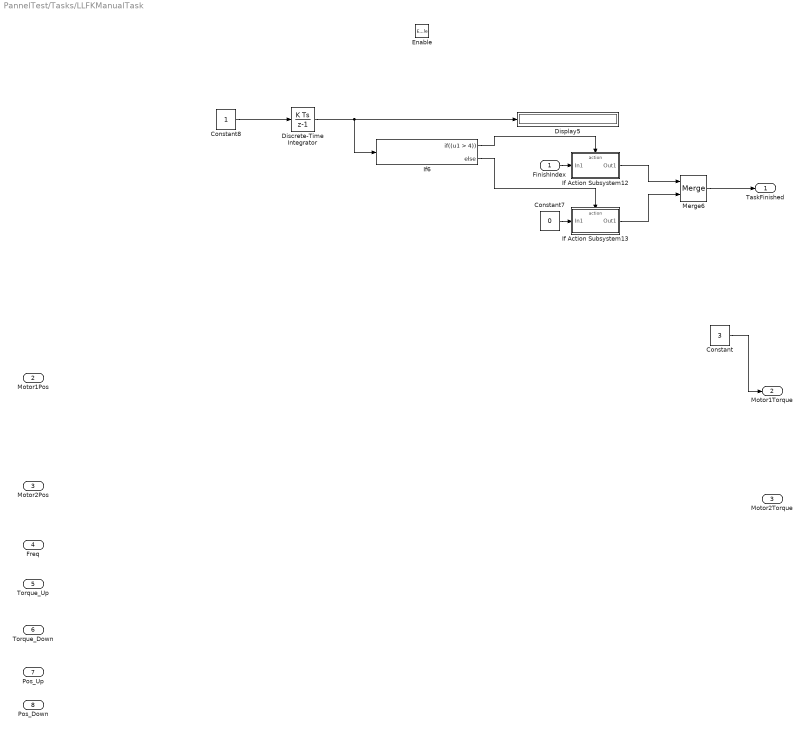
== system PannelTest/Tasks/LLFKManualTask ==
  FinishIndex : Inport
  Motor1Pos : Inport  Port=2
  Motor2Pos : Inport  Port=3
  Freq : Inport  Port=4
  Torque_Up : Inport  Port=5
  Torque_Down : Inport  Port=6
  Pos_Up : Inport  Port=7
  Pos_Down : Inport  Port=8
  Enable : EnablePort  StatesWhenEnabling=reset
  Constant : Constant  Value=3
  Constant7 : Constant  Value=0  OutDataTypeStr=double
  Constant8 : Constant
  Discrete-Time Integrator : DiscreteIntegrator  SampleTime=-1  ICPrevOutput=DiscIntNeverNeededParam  ICPrevScaledInput=DiscIntNeverNeededParam
  Display5 : Display
  If Action Subsystem12 : Subsystem  TreatAsAtomicUnit=on
  If Action Subsystem13 : Subsystem  TreatAsAtomicUnit=on
  If6 : If  IfExpression=(u1 > 4)
  Merge6 : Merge
  TaskFinished : Outport
  Motor1Torque : Outport  Port=2
  Motor2Torque : Outport  Port=3
  wires:
  Merge6/1 -> TaskFinished/1
  If6/1 -> If Action Subsystem12/Action
  Constant8/1 -> Discrete-Time Integrator/1
  If6/2 -> If Action Subsystem13/Action
  Discrete-Time Integrator/1 -> If6/1, Display5/1
  If Action Subsystem13/1(Out1) -> Merge6/2
  FinishIndex/1 -> If Action Subsystem12/1(In1)
  If Action Subsystem12/1(Out1) -> Merge6/1
  Constant7/1 -> If Action Subsystem13/1(In1)
  Constant/1 -> Motor1Torque/1

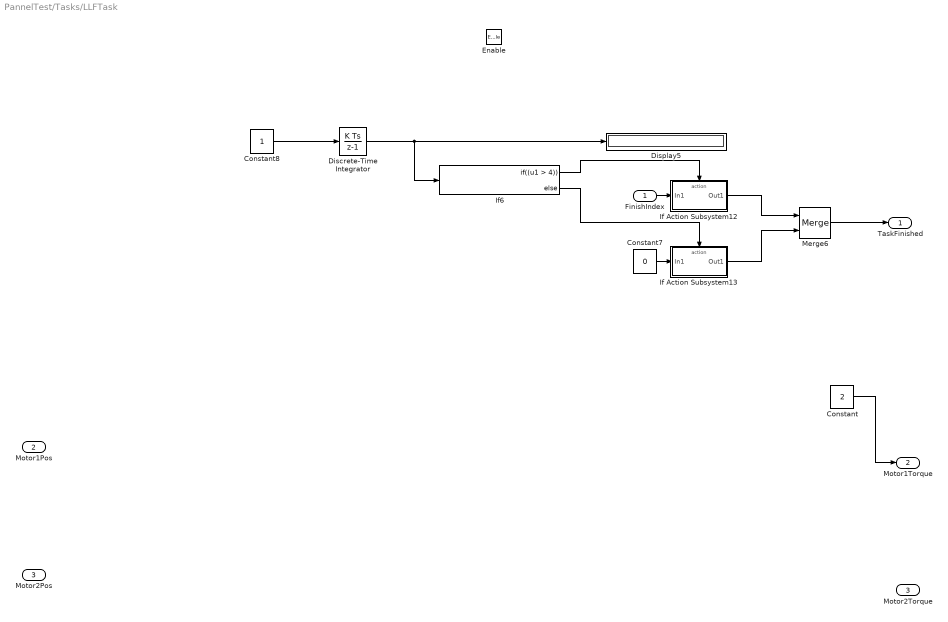
== system PannelTest/Tasks/LLFTask ==
  FinishIndex : Inport
  Motor1Pos : Inport  Port=2
  Motor2Pos : Inport  Port=3
  Enable : EnablePort  StatesWhenEnabling=reset
  Constant : Constant  Value=2
  Constant7 : Constant  Value=0  OutDataTypeStr=double
  Constant8 : Constant
  Discrete-Time Integrator : DiscreteIntegrator  SampleTime=-1  ICPrevOutput=DiscIntNeverNeededParam  ICPrevScaledInput=DiscIntNeverNeededParam
  Display5 : Display
  If Action Subsystem12 : Subsystem  TreatAsAtomicUnit=on
  If Action Subsystem13 : Subsystem  TreatAsAtomicUnit=on
  If6 : If  IfExpression=(u1 > 4)
  Merge6 : Merge
  TaskFinished : Outport
  Motor1Torque : Outport  Port=2
  Motor2Torque : Outport  Port=3
  wires:
  Merge6/1 -> TaskFinished/1
  If6/1 -> If Action Subsystem12/Action
  Constant8/1 -> Discrete-Time Integrator/1
  If6/2 -> If Action Subsystem13/Action
  Discrete-Time Integrator/1 -> If6/1, Display5/1
  If Action Subsystem13/1(Out1) -> Merge6/2
  FinishIndex/1 -> If Action Subsystem12/1(In1)
  If Action Subsystem12/1(Out1) -> Merge6/1
  Constant7/1 -> If Action Subsystem13/1(In1)
  Constant/1 -> Motor1Torque/1

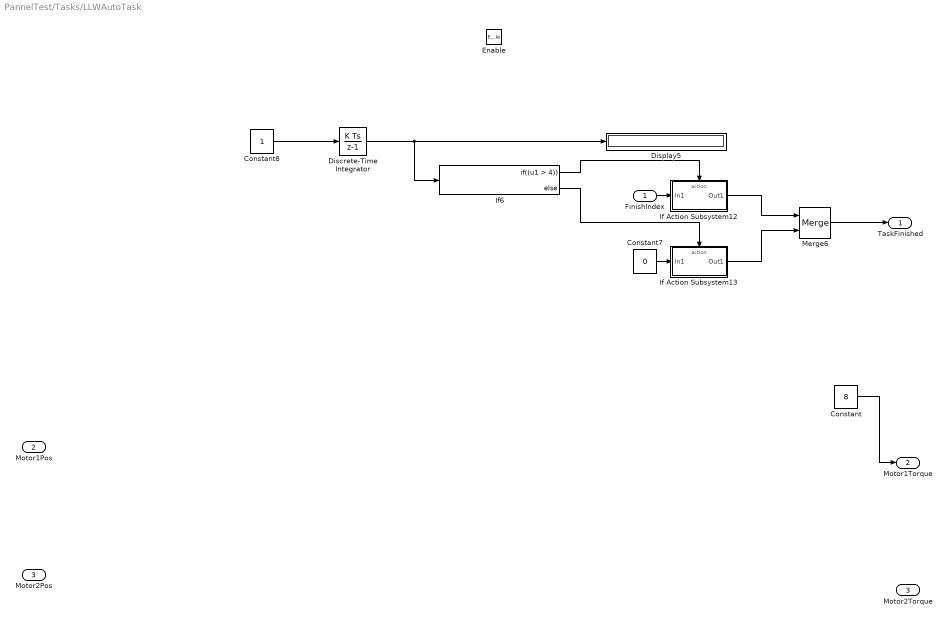
== system PannelTest/Tasks/LLWAutoTask ==
  FinishIndex : Inport
  Motor1Pos : Inport  Port=2
  Motor2Pos : Inport  Port=3
  Enable : EnablePort  StatesWhenEnabling=reset
  Constant : Constant  Value=8
  Constant7 : Constant  Value=0  OutDataTypeStr=double
  Constant8 : Constant
  Discrete-Time Integrator : DiscreteIntegrator  SampleTime=-1  ICPrevOutput=DiscIntNeverNeededParam  ICPrevScaledInput=DiscIntNeverNeededParam
  Display5 : Display
  If Action Subsystem12 : Subsystem  TreatAsAtomicUnit=on
  If Action Subsystem13 : Subsystem  TreatAsAtomicUnit=on
  If6 : If  IfExpression=(u1 > 4)
  Merge6 : Merge
  TaskFinished : Outport
  Motor1Torque : Outport  Port=2
  Motor2Torque : Outport  Port=3
  wires:
  Merge6/1 -> TaskFinished/1
  If6/1 -> If Action Subsystem12/Action
  Constant8/1 -> Discrete-Time Integrator/1
  If6/2 -> If Action Subsystem13/Action
  Discrete-Time Integrator/1 -> If6/1, Display5/1
  If Action Subsystem13/1(Out1) -> Merge6/2
  FinishIndex/1 -> If Action Subsystem12/1(In1)
  If Action Subsystem12/1(Out1) -> Merge6/1
  Constant7/1 -> If Action Subsystem13/1(In1)
  Constant/1 -> Motor1Torque/1

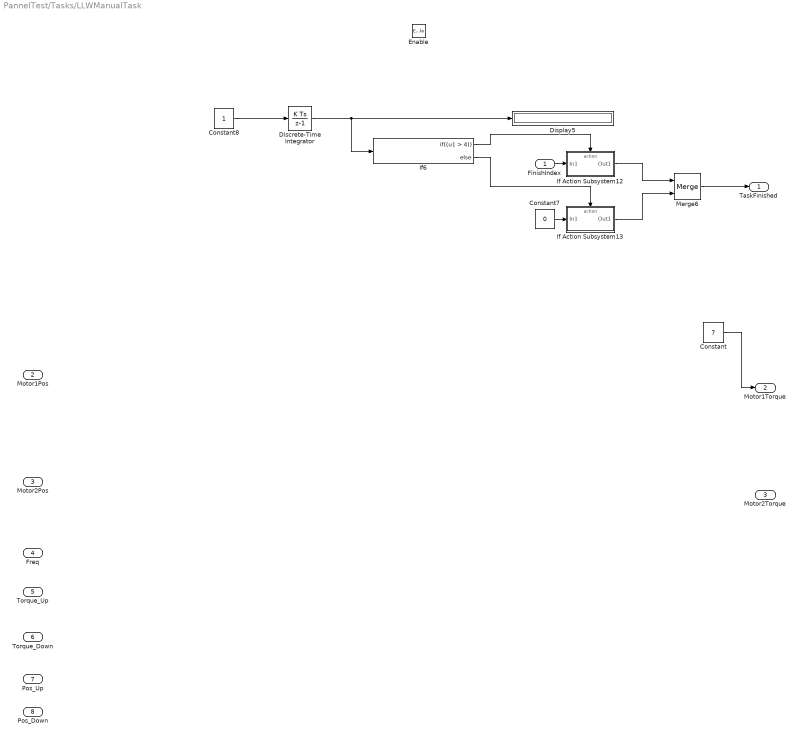
== system PannelTest/Tasks/LLWManualTask ==
  FinishIndex : Inport
  Motor1Pos : Inport  Port=2
  Motor2Pos : Inport  Port=3
  Freq : Inport  Port=4
  Torque_Up : Inport  Port=5
  Torque_Down : Inport  Port=6
  Pos_Up : Inport  Port=7
  Pos_Down : Inport  Port=8
  Enable : EnablePort  StatesWhenEnabling=reset
  Constant : Constant  Value=7
  Constant7 : Constant  Value=0  OutDataTypeStr=double
  Constant8 : Constant
  Discrete-Time Integrator : DiscreteIntegrator  SampleTime=-1  ICPrevOutput=DiscIntNeverNeededParam  ICPrevScaledInput=DiscIntNeverNeededParam
  Display5 : Display
  If Action Subsystem12 : Subsystem  TreatAsAtomicUnit=on
  If Action Subsystem13 : Subsystem  TreatAsAtomicUnit=on
  If6 : If  IfExpression=(u1 > 4)
  Merge6 : Merge
  TaskFinished : Outport
  Motor1Torque : Outport  Port=2
  Motor2Torque : Outport  Port=3
  wires:
  Merge6/1 -> TaskFinished/1
  If6/1 -> If Action Subsystem12/Action
  Constant8/1 -> Discrete-Time Integrator/1
  If6/2 -> If Action Subsystem13/Action
  Discrete-Time Integrator/1 -> If6/1, Display5/1
  If Action Subsystem13/1(Out1) -> Merge6/2
  FinishIndex/1 -> If Action Subsystem12/1(In1)
  If Action Subsystem12/1(Out1) -> Merge6/1
  Constant7/1 -> If Action Subsystem13/1(In1)
  Constant/1 -> Motor1Torque/1

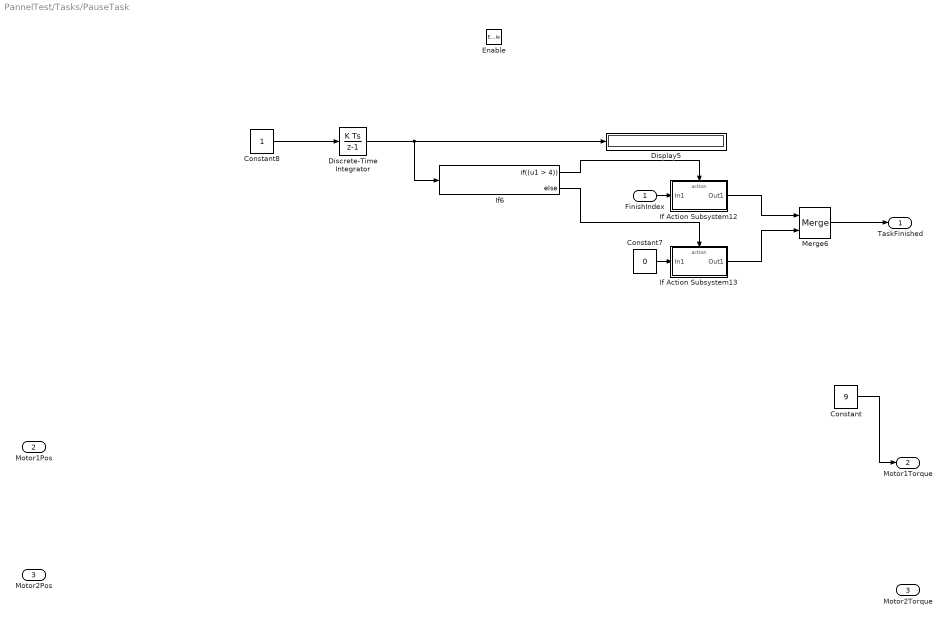
== system PannelTest/Tasks/PauseTask ==
  FinishIndex : Inport
  Motor1Pos : Inport  Port=2
  Motor2Pos : Inport  Port=3
  Enable : EnablePort  StatesWhenEnabling=reset
  Constant : Constant  Value=9
  Constant7 : Constant  Value=0  OutDataTypeStr=double
  Constant8 : Constant
  Discrete-Time Integrator : DiscreteIntegrator  SampleTime=-1  ICPrevOutput=DiscIntNeverNeededParam  ICPrevScaledInput=DiscIntNeverNeededParam
  Display5 : Display
  If Action Subsystem12 : Subsystem  TreatAsAtomicUnit=on
  If Action Subsystem13 : Subsystem  TreatAsAtomicUnit=on
  If6 : If  IfExpression=(u1 > 4)
  Merge6 : Merge
  TaskFinished : Outport
  Motor1Torque : Outport  Port=2
  Motor2Torque : Outport  Port=3
  wires:
  Merge6/1 -> TaskFinished/1
  If6/1 -> If Action Subsystem12/Action
  Constant8/1 -> Discrete-Time Integrator/1
  If6/2 -> If Action Subsystem13/Action
  Discrete-Time Integrator/1 -> If6/1, Display5/1
  If Action Subsystem13/1(Out1) -> Merge6/2
  FinishIndex/1 -> If Action Subsystem12/1(In1)
  If Action Subsystem12/1(Out1) -> Merge6/1
  Constant7/1 -> If Action Subsystem13/1(In1)
  Constant/1 -> Motor1Torque/1

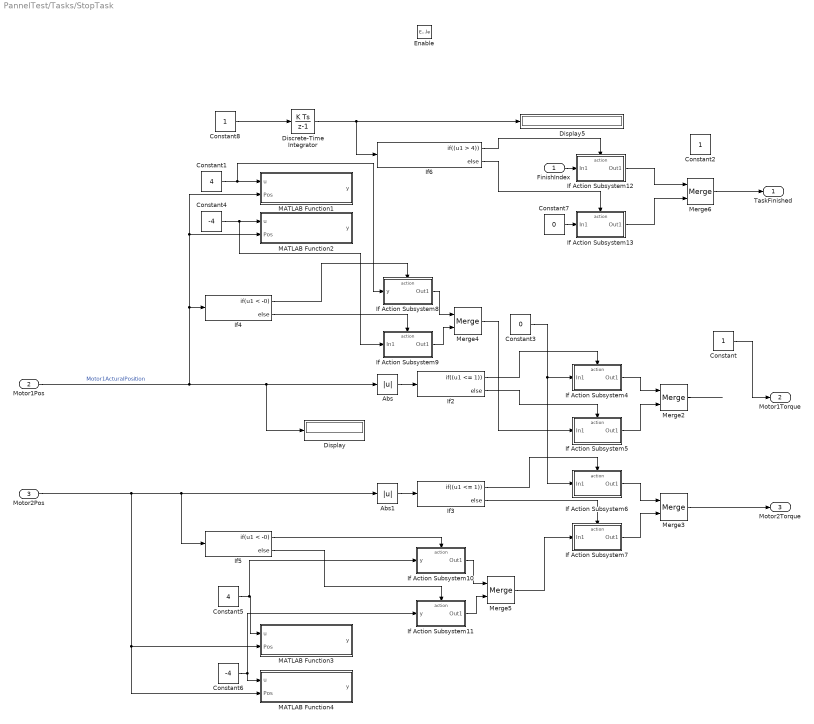
== system PannelTest/Tasks/StopTask ==
  FinishIndex : Inport
  Motor1Pos : Inport  Port=2
  Motor2Pos : Inport  Port=3
  Enable : EnablePort  StatesWhenEnabling=reset
  Abs : Abs  SaturateOnIntegerOverflow=off
  Abs1 : Abs  SaturateOnIntegerOverflow=off
  Constant : Constant
  Constant1 : Constant  Value=4
  Constant2 : Constant
  Constant3 : Constant  Value=0
  Constant4 : Constant  Value=-4
  Constant5 : Constant  Value=4
  Constant6 : Constant  Value=-4
  Constant7 : Constant  Value=0  OutDataTypeStr=double
  Constant8 : Constant
  Discrete-Time Integrator : DiscreteIntegrator  SampleTime=-1  ICPrevOutput=DiscIntNeverNeededParam  ICPrevScaledInput=DiscIntNeverNeededParam
  Display : Display
  Display5 : Display
  If Action Subsystem10 : Subsystem  TreatAsAtomicUnit=on
  If Action Subsystem11 : Subsystem  TreatAsAtomicUnit=on
  If Action Subsystem12 : Subsystem  TreatAsAtomicUnit=on
  If Action Subsystem13 : Subsystem  TreatAsAtomicUnit=on
  If Action Subsystem4 : Subsystem  TreatAsAtomicUnit=on
  If Action Subsystem5 : Subsystem  TreatAsAtomicUnit=on
  If Action Subsystem6 : Subsystem  TreatAsAtomicUnit=on
  If Action Subsystem7 : Subsystem  TreatAsAtomicUnit=on
  If Action Subsystem8 : Subsystem  TreatAsAtomicUnit=on
  If Action Subsystem9 : Subsystem  TreatAsAtomicUnit=on
  If2 : If  IfExpression=(u1 <= 1)
  If3 : If  IfExpression=(u1 <= 1)
  If4 : If  IfExpression=u1 < -0
  If5 : If  IfExpression=u1 < -0
  If6 : If  IfExpression=(u1 > 4)
  MATLAB Function1 : MATLAB Function  TreatAsAtomicUnit=on
  MATLAB Function2 : MATLAB Function  TreatAsAtomicUnit=on
  MATLAB Function3 : MATLAB Function  TreatAsAtomicUnit=on
  MATLAB Function4 : MATLAB Function  TreatAsAtomicUnit=on
  Merge{2..6} (5 alike) : Merge
  TaskFinished : Outport
  Motor1Torque : Outport  Port=2
  Motor2Torque : Outport  Port=3
  wires:
  Merge6/1 -> TaskFinished/1
  If6/1 -> If Action Subsystem12/Action
  If2/1 -> If Action Subsystem4/Action
  Constant1/1 -> If Action Subsystem8/1(y), MATLAB Function1/1(u)
  If Action Subsystem11/1(Out1) -> Merge5/2
  Constant5/1 -> If Action Subsystem10/1(y), MATLAB Function3/1(u)
  If5/2 -> If Action Subsystem11/Action
  If4/2 -> If Action Subsystem9/Action
  If Action Subsystem8/1(Out1) -> Merge4/1
  If3/2 -> If Action Subsystem7/Action
  If4/1 -> If Action Subsystem8/Action
  If Action Subsystem10/1(Out1) -> Merge5/1
  Constant8/1 -> Discrete-Time Integrator/1
  If2/2 -> If Action Subsystem5/Action
  Merge5/1 -> If Action Subsystem7/1(In1)
  Merge3/1 -> Motor2Torque/1
  If5/1 -> If Action Subsystem10/Action
  Abs/1 -> If2/1
  Merge4/1 -> If Action Subsystem5/1(In1)
  Merge2/1 -> ?
  Constant3/1 -> If Action Subsystem6/1(In1), If Action Subsystem4/1(In1)
  If Action Subsystem9/1(Out1) -> Merge4/2
  Motor2Pos/1 -> MATLAB Function4/2(Pos), MATLAB Function3/2(Pos), If5/1, Abs1/1
  Motor1Pos/1 -> MATLAB Function2/2(Pos), MATLAB Function1/2(Pos), If4/1, Abs/1, Display/1  "Motor1ActuralPosition"
  If6/2 -> If Action Subsystem13/Action
  Abs1/1 -> If3/1
  Discrete-Time Integrator/1 -> If6/1, Display5/1
  If Action Subsystem13/1(Out1) -> Merge6/2
  If Action Subsystem7/1(Out1) -> Merge3/2
  FinishIndex/1 -> If Action Subsystem12/1(In1)
  If Action Subsystem12/1(Out1) -> Merge6/1
  If Action Subsystem6/1(Out1) -> Merge3/1
  If Action Subsystem4/1(Out1) -> Merge2/1
  If3/1 -> If Action Subsystem6/Action
  If Action Subsystem5/1(Out1) -> Merge2/2
  Constant7/1 -> If Action Subsystem13/1(In1)
  Constant4/1 -> If Action Subsystem9/1(In1), MATLAB Function2/1(u)
  Constant6/1 -> If Action Subsystem11/1(y), MATLAB Function4/1(u)
  Constant/1 -> Motor1Torque/1

== system PannelTest/Tasks/ULLockTask ==
  FinishIndex : Inport
  Motor3Pos : Inport  Port=2
  Motor4Pos : Inport  Port=3
  Enable : EnablePort  StatesWhenEnabling=reset
  Constant : Constant  Value=2
  Constant7 : Constant  Value=0  OutDataTypeStr=double
  Constant8 : Constant
  Discrete-Time Integrator : DiscreteIntegrator  SampleTime=-1  ICPrevOutput=DiscIntNeverNeededParam  ICPrevScaledInput=DiscIntNeverNeededParam
  Display5 : Display
  If Action Subsystem12 : Subsystem  TreatAsAtomicUnit=on
  If Action Subsystem13 : Subsystem  TreatAsAtomicUnit=on
  If6 : If  IfExpression=(u1 > 4)
  Merge6 : Merge
  TaskFinished : Outport
  Motor3Torque : Outport  Port=2
  Motor4Torque : Outport  Port=3
  wires:
  Merge6/1 -> TaskFinished/1
  If6/1 -> If Action Subsystem12/Action
  Constant8/1 -> Discrete-Time Integrator/1
  If6/2 -> If Action Subsystem13/Action
  Discrete-Time Integrator/1 -> If6/1, Display5/1
  If Action Subsystem13/1(Out1) -> Merge6/2
  FinishIndex/1 -> If Action Subsystem12/1(In1)
  If Action Subsystem12/1(Out1) -> Merge6/1
  Constant7/1 -> If Action Subsystem13/1(In1)
  Constant/1 -> Motor3Torque/1

== system PannelTest/Tasks/ULUnLockTask ==
  FinishIndex : Inport
  Motor3Pos : Inport  Port=2
  Motor4Pos : Inport  Port=3
  Enable : EnablePort  StatesWhenEnabling=reset
  Constant : Constant
  Constant7 : Constant  Value=0  OutDataTypeStr=double
  Constant8 : Constant
  Discrete-Time Integrator : DiscreteIntegrator  SampleTime=-1  ICPrevOutput=DiscIntNeverNeededParam  ICPrevScaledInput=DiscIntNeverNeededParam
  Display5 : Display
  If Action Subsystem12 : Subsystem  TreatAsAtomicUnit=on
  If Action Subsystem13 : Subsystem  TreatAsAtomicUnit=on
  If6 : If  IfExpression=(u1 > 4)
  Merge6 : Merge
  TaskFinished : Outport
  Motor3Torque : Outport  Port=2
  Motor4Torque : Outport  Port=3
  wires:
  Merge6/1 -> TaskFinished/1
  If6/1 -> If Action Subsystem12/Action
  Constant8/1 -> Discrete-Time Integrator/1
  If6/2 -> If Action Subsystem13/Action
  Discrete-Time Integrator/1 -> If6/1, Display5/1
  If Action Subsystem13/1(Out1) -> Merge6/2
  FinishIndex/1 -> If Action Subsystem12/1(In1)
  If Action Subsystem12/1(Out1) -> Merge6/1
  Constant7/1 -> If Action Subsystem13/1(In1)
  Constant/1 -> Motor3Torque/1

== system PannelTest/PanelController/Display_State_1_Enable/Subsystem ==
  Case : Inport
  Case Default : Inport  Port=2
  Constant : Constant
  Constant1 : Constant  Value=0
  Constant2 : Constant  Value=TaskIndex
  Merge : Merge
  Switch Case Action Subsystem : Subsystem  TreatAsAtomicUnit=on
  Switch Case Action Subsystem1 : Subsystem  TreatAsAtomicUnit=on
  Enable : Outport
  FinishIndex : Outport  Port=2
  wires:
  Constant/1 -> Switch Case Action Subsystem/1(In1)
  Case/1 -> Switch Case Action Subsystem/Action
  Switch Case Action Subsystem/1(Out1) -> Merge/1
  Merge/1 -> Enable/1
  Case Default/1 -> Switch Case Action Subsystem1/Action
  Constant1/1 -> Switch Case Action Subsystem1/1(In1)
  Switch Case Action Subsystem1/1(Default) -> Merge/2
  Constant2/1 -> FinishIndex/1

== system PannelTest/PanelController/Display_State_2_Enable/Subsystem ==
  Case : Inport
  Case Default : Inport  Port=2
  Constant : Constant
  Constant1 : Constant  Value=0
  Constant2 : Constant  Value=TaskIndex
  Merge : Merge
  Switch Case Action Subsystem : Subsystem  TreatAsAtomicUnit=on
  Switch Case Action Subsystem1 : Subsystem  TreatAsAtomicUnit=on
  Enable : Outport
  FinishIndex : Outport  Port=2
  wires:
  Constant/1 -> Switch Case Action Subsystem/1(In1)
  Case/1 -> Switch Case Action Subsystem/Action
  Switch Case Action Subsystem/1(Out1) -> Merge/1
  Merge/1 -> Enable/1
  Case Default/1 -> Switch Case Action Subsystem1/Action
  Constant1/1 -> Switch Case Action Subsystem1/1(In1)
  Switch Case Action Subsystem1/1(Default) -> Merge/2
  Constant2/1 -> FinishIndex/1

== system PannelTest/PanelController/Display_State_3_Enable/Subsystem ==
  Case : Inport
  Case Default : Inport  Port=2
  Constant : Constant
  Constant1 : Constant  Value=0
  Constant2 : Constant  Value=TaskIndex
  Merge : Merge
  Switch Case Action Subsystem : Subsystem  TreatAsAtomicUnit=on
  Switch Case Action Subsystem1 : Subsystem  TreatAsAtomicUnit=on
  Enable : Outport
  FinishIndex : Outport  Port=2
  wires:
  Constant/1 -> Switch Case Action Subsystem/1(In1)
  Case/1 -> Switch Case Action Subsystem/Action
  Switch Case Action Subsystem/1(Out1) -> Merge/1
  Merge/1 -> Enable/1
  Case Default/1 -> Switch Case Action Subsystem1/Action
  Constant1/1 -> Switch Case Action Subsystem1/1(In1)
  Switch Case Action Subsystem1/1(Default) -> Merge/2
  Constant2/1 -> FinishIndex/1
